simulink model "IpSDKSebesegEsPozicio"  (R2013b)
settings: Solver=FixedStepDiscrete  SolverMode=SingleTasking  StartTime=0.0  StopTime=10.0  FixedStep=1  RelTol=1e-3
undefined symbols (not defined in the file or in its folder): gcbh, xlBlockLoadCallback, xlGetNormalizedPeriod
libraries: xbsIndex_r4 x250
(part 2 of 2)

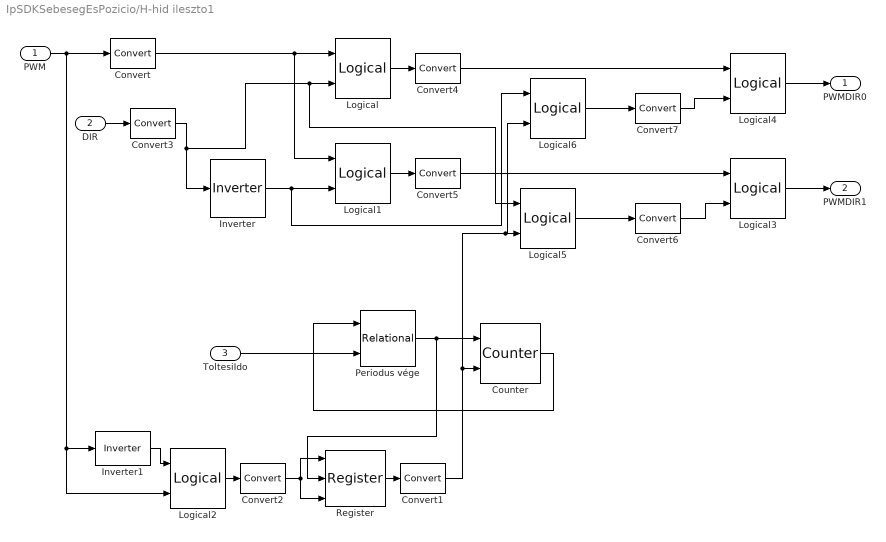
== system IpSDKSebesegEsPozicio/H-hid ileszto1 ==
  PWM : Inport
  DIR : Inport  Port=2
  ToltesiIdo : Inport  Port=3
  Convert{,1..7} (8 alike) : xbsIndex_r4/Convert  gui_display_data_type=Boolean  arith_type=Boolean  n_bits=16  bin_pt=14  float_type=Single  exp_bits=8  fraction_bits=24  quantization=Truncate  overflow=Wrap  en=off  latency=0  dbl_ovrd=off  pipeline=off  block_type=convert
  Counter : xbsIndex_r4/Counter  cnt_type=Free Running  cnt_to=Inf  operation=Up  start_count=0  cnt_by_val=1  arith_type=Unsigned  n_bits=16  bin_pt=0  load_pin=off  rst=on  en=on  explicit_period=off  period=2*10^-2  dbl_ovrd=off  use_behavioral_HDL=off  implementation=Fabric  block_type=counter
  Inverter : xbsIndex_r4/Inverter  en=off  latency=0  dbl_ovrd=off  block_type=inv
  Inverter1 : xbsIndex_r4/Inverter  en=off  latency=1  dbl_ovrd=off  block_type=inv
  Logical{,1..2,5..6} (5 alike) : xbsIndex_r4/Logical  logical_function=AND  inputs=2  en=off  latency=0  precision=User Defined  arith_type=Unsigned  n_bits=1  bin_pt=0  align_bp=on  dbl_ovrd=off  block_type=logical
  Logical3 : xbsIndex_r4/Logical  logical_function=OR  inputs=2  en=off  latency=0  precision=User Defined  arith_type=Unsigned  n_bits=1  bin_pt=0  align_bp=on  dbl_ovrd=off  block_type=logical
  Logical4 : xbsIndex_r4/Logical  logical_function=OR  inputs=2  en=off  latency=0  precision=User Defined  arith_type=Unsigned  n_bits=1  bin_pt=0  align_bp=on  dbl_ovrd=off  block_type=logical
  Periodus vége : xbsIndex_r4/Relational  mode=a=b  en=off  latency=0  dbl_ovrd=off  block_type=relational
  Register : xbsIndex_r4/Register  init=0  rst=on  en=on  dbl_ovrd=off  block_type=register
  PWMDIR0 : Outport
  PWMDIR1 : Outport  Port=2
  wires:
  DIR/1 -> Convert3/1
  Inverter/1 -> Logical6/1, Logical1/2
  Convert/1 -> Logical1/1, Logical/1
  Counter/1 -> Periodus vége/1
  Periodus vége/1 -> Register/2, Counter/1
  ToltesiIdo/1 -> Periodus vége/2
  PWM/1 -> Convert/1, Logical2/2, Inverter1/1
  Inverter1/1 -> Logical2/1
  Logical2/1 -> Convert2/1
  Logical3/1 -> PWMDIR1/1
  Logical1/1 -> Convert5/1
  Logical4/1 -> PWMDIR0/1
  Logical/1 -> Convert4/1
  Register/1 -> Convert1/1
  Convert1/1 -> Logical6/2, Logical5/2, Counter/2
  Convert2/1 -> Register/3, Register/1
  Convert3/1 -> Inverter/1, Logical5/1, Logical/2
  Convert4/1 -> Logical4/1
  Convert5/1 -> Logical3/1
  Logical5/1 -> Convert6/1
  Logical6/1 -> Convert7/1
  Convert6/1 -> Logical3/2
  Convert7/1 -> Logical4/2

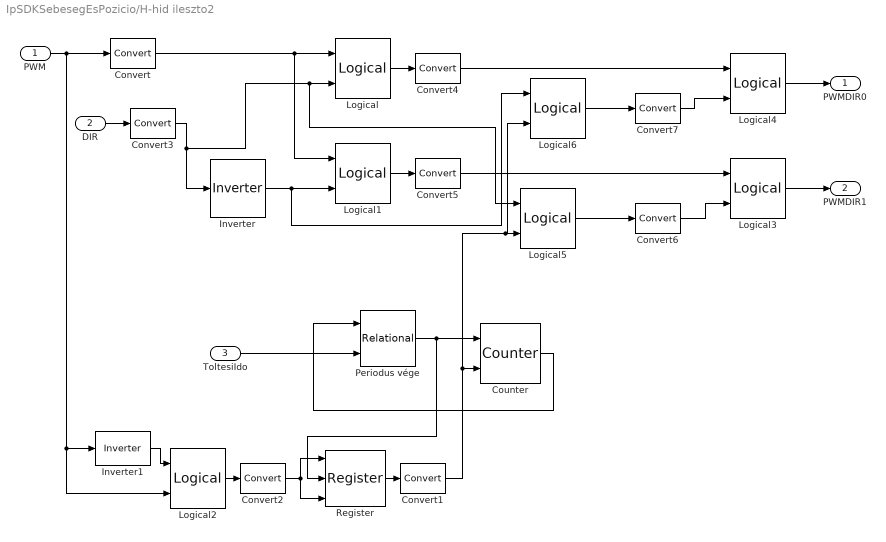
== system IpSDKSebesegEsPozicio/H-hid ileszto2 ==
  PWM : Inport
  DIR : Inport  Port=2
  ToltesiIdo : Inport  Port=3
  Convert{,1..7} (8 alike) : xbsIndex_r4/Convert  gui_display_data_type=Boolean  arith_type=Boolean  n_bits=16  bin_pt=14  float_type=Single  exp_bits=8  fraction_bits=24  quantization=Truncate  overflow=Wrap  en=off  latency=0  dbl_ovrd=off  pipeline=off  block_type=convert
  Counter : xbsIndex_r4/Counter  cnt_type=Free Running  cnt_to=Inf  operation=Up  start_count=0  cnt_by_val=1  arith_type=Unsigned  n_bits=16  bin_pt=0  load_pin=off  rst=on  en=on  explicit_period=off  period=2*10^-2  dbl_ovrd=off  use_behavioral_HDL=off  implementation=Fabric  block_type=counter
  Inverter : xbsIndex_r4/Inverter  en=off  latency=0  dbl_ovrd=off  block_type=inv
  Inverter1 : xbsIndex_r4/Inverter  en=off  latency=1  dbl_ovrd=off  block_type=inv
  Logical{,1..2,5..6} (5 alike) : xbsIndex_r4/Logical  logical_function=AND  inputs=2  en=off  latency=0  precision=User Defined  arith_type=Unsigned  n_bits=1  bin_pt=0  align_bp=on  dbl_ovrd=off  block_type=logical
  Logical3 : xbsIndex_r4/Logical  logical_function=OR  inputs=2  en=off  latency=0  precision=User Defined  arith_type=Unsigned  n_bits=1  bin_pt=0  align_bp=on  dbl_ovrd=off  block_type=logical
  Logical4 : xbsIndex_r4/Logical  logical_function=OR  inputs=2  en=off  latency=0  precision=User Defined  arith_type=Unsigned  n_bits=1  bin_pt=0  align_bp=on  dbl_ovrd=off  block_type=logical
  Periodus vége : xbsIndex_r4/Relational  mode=a=b  en=off  latency=0  dbl_ovrd=off  block_type=relational
  Register : xbsIndex_r4/Register  init=0  rst=on  en=on  dbl_ovrd=off  block_type=register
  PWMDIR0 : Outport
  PWMDIR1 : Outport  Port=2
  wires:
  DIR/1 -> Convert3/1
  Inverter/1 -> Logical6/1, Logical1/2
  Convert/1 -> Logical1/1, Logical/1
  Counter/1 -> Periodus vége/1
  Periodus vége/1 -> Register/2, Counter/1
  ToltesiIdo/1 -> Periodus vége/2
  PWM/1 -> Convert/1, Logical2/2, Inverter1/1
  Inverter1/1 -> Logical2/1
  Logical2/1 -> Convert2/1
  Logical3/1 -> PWMDIR1/1
  Logical1/1 -> Convert5/1
  Logical4/1 -> PWMDIR0/1
  Logical/1 -> Convert4/1
  Register/1 -> Convert1/1
  Convert1/1 -> Logical6/2, Logical5/2, Counter/2
  Convert2/1 -> Register/3, Register/1
  Convert3/1 -> Inverter/1, Logical5/1, Logical/2
  Convert4/1 -> Logical4/1
  Convert5/1 -> Logical3/1
  Logical5/1 -> Convert6/1
  Logical6/1 -> Convert7/1
  Convert6/1 -> Logical3/2
  Convert7/1 -> Logical4/2

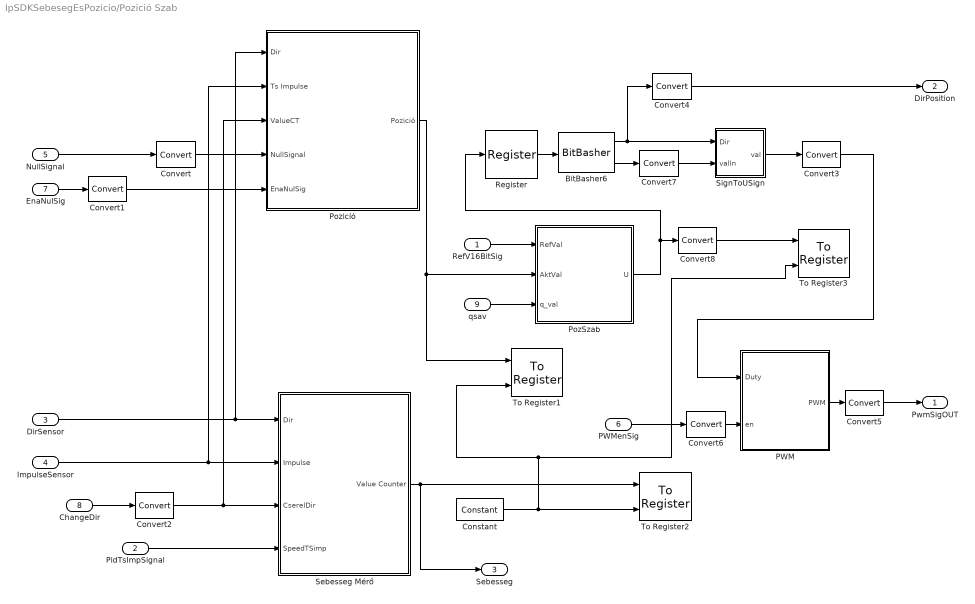
== system IpSDKSebesegEsPozicio/Pozició Szab ==
  RefV16BitSig : Inport
  PidTsImpSignal : Inport  Port=2
  DirSensor : Inport  Port=3
  ImpulseSensor : Inport  Port=4
  NullSignal : Inport  Port=5
  PWMenSig : Inport  Port=6
  EnaNulSig : Inport  Port=7
  ChangeDir : Inport  Port=8
  qsav : Inport  Port=9
  BitBasher6 : xbsIndex_r4/BitBasher  bitexpr=|  display_expr=off  sr_1=1  arith_type1=Unsigned  bin_pt1=0  sr_2=2  arith_type2="Signed  (2's comp)"  bin_pt2=0  sr_3=3  arith_type3=Unsigned  bin_pt3=0  sr_4=4  arith_type4=Unsigned  bin_pt4=0  dbl_ovrd=off  block_type=bitbasher
      | <!DOCTYPE HTML PUBLIC "-//W3C//DTD HTML 4.0//EN" "http://www.w3.org/TR/REC-html40/strict.dtd">
      | <html><head><meta name="qrichtext" content="1" /><style type="text/css">
      | p, li { white-space: pre-wrap; }
      | </style></head><body style=" font-family:'MS Shell Dlg 2'; font-size:8.25pt; font-weight:400; font-style:normal;">
      | <p style=" margin-top:12px; margin-bottom:12px; margin-left:0px; margin-right:0px; -qt-block-indent:0; text-indent:0px;"><span style=" font-family:'MS Shell Dlg'; font-size:8pt;">dir={a[16]}<br />val={a[15:0]}</span></p></body></html>
  Constant : xbsIndex_r4/Constant  const=1  gui_display_data_type=Boolean  arith_type=Boolean  n_bits=16  bin_pt=14  preci_type=Single  exp_width=8  frac_width=24  explicit_period=off  period=1  equ=P=C  opselect=C  inp2=PCIN>>17  opr=+  inp1=P  carry=CIN  dbl_ovrd=off  block_type=constant
  Convert{,1..2,6} (4 alike) : xbsIndex_r4/Convert  gui_display_data_type=Boolean  arith_type=Boolean  n_bits=16  bin_pt=14  float_type=Single  exp_bits=8  fraction_bits=24  quantization=Truncate  overflow=Wrap  en=off  latency=0  dbl_ovrd=off  pipeline=off  block_type=convert
  Convert3 : xbsIndex_r4/Convert  gui_display_data_type=Fixed-point  arith_type=Unsigned  n_bits=16  bin_pt=0  float_type=Single  exp_bits=8  fraction_bits=24  quantization=Truncate  overflow=Wrap  en=off  latency=0  dbl_ovrd=off  pipeline=off  block_type=convert
  Convert4 : xbsIndex_r4/Convert  gui_display_data_type=Boolean  arith_type=Boolean  n_bits=16  bin_pt=0  float_type=Single  exp_bits=8  fraction_bits=24  quantization=Truncate  overflow=Wrap  en=off  latency=0  dbl_ovrd=off  pipeline=off  block_type=convert
  Convert5 : xbsIndex_r4/Convert  gui_display_data_type=Boolean  arith_type=Boolean  n_bits=17  bin_pt=0  float_type=Single  exp_bits=8  fraction_bits=24  quantization=Truncate  overflow=Wrap  en=off  latency=0  dbl_ovrd=off  pipeline=off  block_type=convert
  Convert7 : xbsIndex_r4/Convert  gui_display_data_type=Fixed-point  arith_type=Unsigned  n_bits=16  bin_pt=0  float_type=Single  exp_bits=8  fraction_bits=24  quantization=Truncate  overflow=Wrap  en=off  latency=0  dbl_ovrd=off  pipeline=off  block_type=convert
  Convert8 : xbsIndex_r4/Convert  gui_display_data_type=Fixed-point  arith_type="Signed  (2's comp)"  n_bits=32  bin_pt=0  float_type=Single  exp_bits=8  fraction_bits=24  quantization=Truncate  overflow=Wrap  en=off  latency=0  dbl_ovrd=off  pipeline=off  block_type=convert
  PWM : Subsystem
  PozSzab : Subsystem
  Pozicíó : Subsystem
  Register : xbsIndex_r4/Register  init=0  rst=off  en=off  dbl_ovrd=off  block_type=register
  Sebesseg Mérő : Subsystem
  SignToUSign : Subsystem
  To Register1 : xbsIndex_r4/To Register  shared_memory_name='AktPozicio'  init=0  ownership=Locally owned and initialized  explicit_data_type=on  gui_display_data_type=Fixed-point  arith_type="Signed  (2's comp)"  n_bits=16  bin_pt=0  preci_type=Single  dbl_ovrd=off  block_type=toreg
      settings: AttributesFormatString=<< %<shared_memory_name> >>  infoedit="Register block that writes data to a shared memory register.  Delay of one sample period."
  To Register2 : xbsIndex_r4/To Register  shared_memory_name='SebessegPozicio'  init=0  ownership=Locally owned and initialized  explicit_data_type=on  gui_display_data_type=Fixed-point  arith_type="Signed  (2's comp)"  n_bits=16  bin_pt=0  preci_type=Single  dbl_ovrd=off  block_type=toreg
      settings: AttributesFormatString=<< %<shared_memory_name> >>  infoedit="Register block that writes data to a shared memory register.  Delay of one sample period."
  To Register3 : xbsIndex_r4/To Register  shared_memory_name='UPozicio'  init=0  ownership=Locally owned and initialized  explicit_data_type=on  gui_display_data_type=Fixed-point  arith_type="Signed  (2's comp)"  n_bits=32  bin_pt=0  preci_type=Single  dbl_ovrd=off  block_type=toreg
      settings: AttributesFormatString=<< %<shared_memory_name> >>  infoedit="Register block that writes data to a shared memory register.  Delay of one sample period."  xl_use_area=on  xl_area=[100,0,0,0,0,0,0]
  PwmSigOUT : Outport
  DirPosition : Outport  Port=2
  Sebesseg : Outport  Port=3
  wires:
  PWM/1(PWM) -> Convert5/1
  BitBasher6/1 -> SignToUSign/1(Dir), Convert4/1
  BitBasher6/2 -> Convert7/1
  SignToUSign/1(val) -> Convert3/1
  PozSzab/1(U) -> Register/1, Convert8/1
  Convert3/1 -> PWM/1(Duty)
  Convert7/1 -> SignToUSign/2(valIn)
  RefV16BitSig/1 -> PozSzab/1(RefVal)
  PWMenSig/1 -> Convert6/1
  Convert5/1 -> PwmSigOUT/1
  NullSignal/1 -> Convert/1
  EnaNulSig/1 -> Convert1/1
  Convert4/1 -> DirPosition/1
  ChangeDir/1 -> Convert2/1
  Pozicíó/1(Pozició) -> To Register1/1, PozSzab/2(AktVal)
  qsav/1 -> PozSzab/3(q_val)
  Sebesseg Mérő/1(Value Counter) -> To Register2/1, Sebesseg/1
  Constant/1 -> To Register3/2, To Register1/2, To Register2/2
  Convert8/1 -> To Register3/1
  PidTsImpSignal/1 -> Sebesseg Mérő/4(SpeedTSimp)
  Register/1 -> BitBasher6/1
  Convert/1 -> Pozicíó/4(NullSignal)
  Convert1/1 -> Pozicíó/5(EnaNulSig)
  DirSensor/1 -> Pozicíó/1(Dir), Sebesseg Mérő/1(Dir)
  ImpulseSensor/1 -> Pozicíó/2(Ts Impulse), Sebesseg Mérő/2(Impulse)
  Convert2/1 -> Pozicíó/3(ValueCT), Sebesseg Mérő/3(CserelDir)
  Convert6/1 -> PWM/2(en)

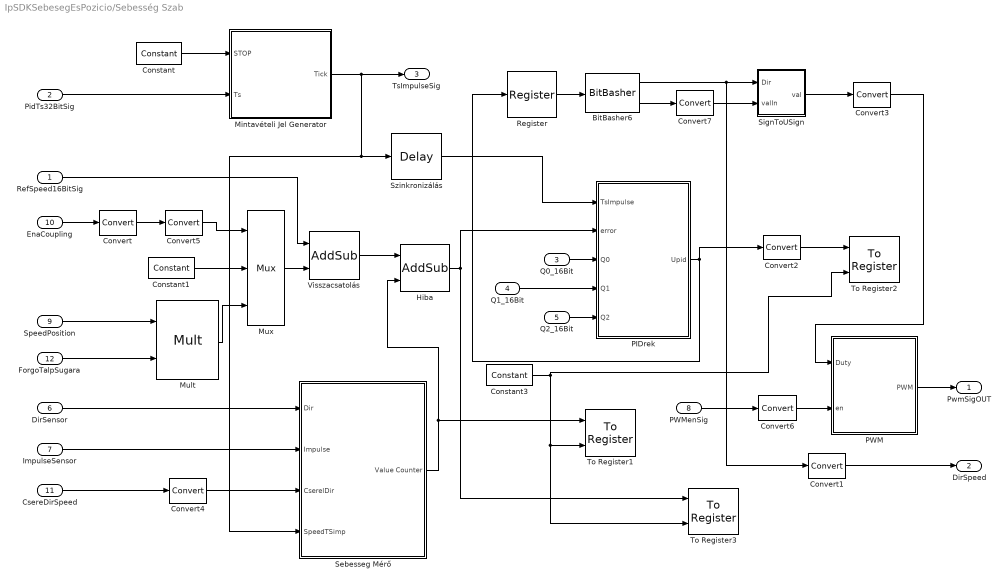
== system IpSDKSebesegEsPozicio/Sebesség Szab ==
  RefSpeed16BitSig : Inport
  PidTs32BitSig : Inport  Port=2
  Q0_16Bit : Inport  Port=3
  Q1_16Bit : Inport  Port=4
  Q2_16Bit : Inport  Port=5
  DirSensor : Inport  Port=6
  ImpulseSensor : Inport  Port=7
  PWMenSig : Inport  Port=8
  SpeedPosition : Inport  Port=9
  EnaCoupling : Inport  Port=10
  CsereDirSpeed : Inport  Port=11
  ForgoTalpSugara : Inport  Port=12
  BitBasher6 : xbsIndex_r4/BitBasher  bitexpr=|  display_expr=off  sr_1=1  arith_type1=Unsigned  bin_pt1=0  sr_2=2  arith_type2=Unsigned  bin_pt2=0  sr_3=3  arith_type3=Unsigned  bin_pt3=0  sr_4=4  arith_type4=Unsigned  bin_pt4=0  dbl_ovrd=off  block_type=bitbasher
      | <!DOCTYPE HTML PUBLIC "-//W3C//DTD HTML 4.0//EN" "http://www.w3.org/TR/REC-html40/strict.dtd">
      | <html><head><meta name="qrichtext" content="1" /><style type="text/css">
      | p, li { white-space: pre-wrap; }
      | </style></head><body style=" font-family:'MS Shell Dlg 2'; font-size:8.25pt; font-weight:400; font-style:normal;">
      | <p style=" margin-top:12px; margin-bottom:12px; margin-left:0px; margin-right:0px; -qt-block-indent:0; text-indent:0px;"><span style=" font-family:'MS Shell Dlg'; font-size:8pt;">dir={a[16]}<br />val={a[15:0]}</span></p></body></html>
  Constant : xbsIndex_r4/Constant  const=0  gui_display_data_type=Boolean  arith_type=Boolean  n_bits=16  bin_pt=14  preci_type=Single  exp_width=8  frac_width=24  explicit_period=off  period=1  equ=P=C  opselect=C  inp2=PCIN>>17  opr=+  inp1=P  carry=CIN  dbl_ovrd=off  block_type=constant
  Constant1 : xbsIndex_r4/Constant  const=0  gui_display_data_type=Fixed-point  arith_type=Signed (2's comp)  n_bits=16  bin_pt=0  preci_type=Single  exp_width=8  frac_width=24  explicit_period=off  period=1  equ=P=C  opselect=C  inp2=PCIN>>17  opr=+  inp1=P  carry=CIN  dbl_ovrd=off  block_type=constant
  Constant3 : xbsIndex_r4/Constant  const=1  gui_display_data_type=Boolean  arith_type=Boolean  n_bits=16  bin_pt=14  preci_type=Single  exp_width=8  frac_width=24  explicit_period=off  period=1  equ=P=C  opselect=C  inp2=PCIN>>17  opr=+  inp1=P  carry=CIN  dbl_ovrd=off  block_type=constant
  Convert{,4..6} (4 alike) : xbsIndex_r4/Convert  gui_display_data_type=Boolean  arith_type=Boolean  n_bits=16  bin_pt=14  float_type=Single  exp_bits=8  fraction_bits=24  quantization=Truncate  overflow=Wrap  en=off  latency=0  dbl_ovrd=off  pipeline=off  block_type=convert
  Convert1 : xbsIndex_r4/Convert  gui_display_data_type=Boolean  arith_type=Boolean  n_bits=16  bin_pt=0  float_type=Single  exp_bits=8  fraction_bits=24  quantization=Truncate  overflow=Wrap  en=off  latency=0  dbl_ovrd=off  pipeline=off  block_type=convert
  Convert2 : xbsIndex_r4/Convert  gui_display_data_type=Fixed-point  arith_type="Signed  (2's comp)"  n_bits=32  bin_pt=0  float_type=Single  exp_bits=8  fraction_bits=24  quantization=Truncate  overflow=Saturate  en=off  latency=0  dbl_ovrd=off  pipeline=off  block_type=convert
  Convert3 : xbsIndex_r4/Convert  gui_display_data_type=Fixed-point  arith_type=Unsigned  n_bits=16  bin_pt=0  float_type=Single  exp_bits=8  fraction_bits=24  quantization=Truncate  overflow=Wrap  en=off  latency=0  dbl_ovrd=off  pipeline=off  block_type=convert
  Convert7 : xbsIndex_r4/Convert  gui_display_data_type=Fixed-point  arith_type=Unsigned  n_bits=16  bin_pt=0  float_type=Single  exp_bits=8  fraction_bits=24  quantization=Truncate  overflow=Wrap  en=off  latency=0  dbl_ovrd=off  pipeline=off  block_type=convert
  Hiba : xbsIndex_r4/AddSub  mode=Subtraction  use_carryin=off  use_carryout=off  en=off  latency=0  precision=User Defined  arith_type="Signed  (2's comp)"  n_bits=16  bin_pt=0  quantization=Truncate  overflow=Saturate  dbl_ovrd=off  use_behavioral_HDL=off  hw_selection=Fabric  pipelined=off  block_type=addsub
      settings: xl_area=[10,0,0,0,0,0,0]
  Mintavételi Jel Generator : Subsystem
  Mult : xbsIndex_r4/Mult  precision=User Defined  arith_type="Signed  (2's comp)"  n_bits=16  bin_pt=0  quantization=Truncate  overflow=Saturate  en=off  latency=3  dbl_ovrd=off  use_behavioral_HDL=off  opt=Area  use_embedded=on  optimum_pipeline=off  pipeline=on  use_rpm=on  placement_style=Triangular  block_type=mult
  Mux : xbsIndex_r4/Mux  inputs=2  en=off  latency=0  precision=User Defined  arith_type="Signed  (2's comp)"  n_bits=16  bin_pt=0  quantization=Truncate  overflow=Saturate  dbl_ovrd=off  block_type=mux
      settings: xl_use_area=on  xl_area=[1,0,0,0,0,0,0]
  PIDrek : Subsystem
  PWM : Subsystem
  Register : xbsIndex_r4/Register  init=0  rst=off  en=off  dbl_ovrd=off  block_type=register
  Sebesseg Mérő : Subsystem
  SignToUSign : Subsystem
  Szinkronizálás : xbsIndex_r4/Delay  rst=off  infoeditControl=Selection of Reset will increase slice count due to use of real FFs and instead of SRLs  en=off  latency=6  dbl_ovrd=off  reg_retiming=off  block_type=delay
      settings: xl_area=[10,0,0,0,0,0,0]
  To Register1 : xbsIndex_r4/To Register  shared_memory_name='AktSebesseg'  init=0  ownership=Locally owned and initialized  explicit_data_type=on  gui_display_data_type=Fixed-point  arith_type="Signed  (2's comp)"  n_bits=16  bin_pt=0  preci_type=Single  dbl_ovrd=off  block_type=toreg
      settings: AttributesFormatString=<< %<shared_memory_name> >>  infoedit="Register block that writes data to a shared memory register.  Delay of one sample period."
  To Register2 : xbsIndex_r4/To Register  shared_memory_name='USebesseg'  init=0  ownership=Locally owned and initialized  explicit_data_type=on  gui_display_data_type=Fixed-point  arith_type="Signed  (2's comp)"  n_bits=32  bin_pt=0  preci_type=Single  dbl_ovrd=off  block_type=toreg
      settings: AttributesFormatString=<< %<shared_memory_name> >>  infoedit="Register block that writes data to a shared memory register.  Delay of one sample period."
  To Register3 : xbsIndex_r4/To Register  shared_memory_name='eSebesseg'  init=0  ownership=Locally owned and initialized  explicit_data_type=on  gui_display_data_type=Fixed-point  arith_type="Signed  (2's comp)"  n_bits=16  bin_pt=0  preci_type=Single  dbl_ovrd=off  block_type=toreg
      settings: AttributesFormatString=<< %<shared_memory_name> >>  infoedit="Register block that writes data to a shared memory register.  Delay of one sample period."
  Visszacsatolás : xbsIndex_r4/AddSub  mode=Subtraction  use_carryin=off  use_carryout=off  en=off  latency=0  precision=User Defined  arith_type="Signed  (2's comp)"  n_bits=16  bin_pt=0  quantization=Truncate  overflow=Saturate  dbl_ovrd=off  use_behavioral_HDL=off  hw_selection=Fabric  pipelined=off  block_type=addsub
  PwmSigOUT : Outport
  DirSpeed : Outport  Port=2
  TsImpulseSig : Outport  Port=3
  wires:
  BitBasher6/1 -> SignToUSign/1(Dir), Convert1/1
  BitBasher6/2 -> Convert7/1
  SignToUSign/1(val) -> Convert3/1
  PIDrek/1(Upid) -> Convert2/1, Register/1
  Convert3/1 -> PWM/1(Duty)
  Convert7/1 -> SignToUSign/2(valIn)
  Mintavételi Jel Generator/1(Tick) -> TsImpulseSig/1, Szinkronizálás/1, Sebesseg Mérő/4(SpeedTSimp)
  Constant/1 -> Mintavételi Jel Generator/1(STOP)
  Szinkronizálás/1 -> PIDrek/1(TsImpulse)
  PidTs32BitSig/1 -> Mintavételi Jel Generator/2(Ts)
  Q2_16Bit/1 -> PIDrek/5(Q2)
  Q1_16Bit/1 -> PIDrek/4(Q1)
  Q0_16Bit/1 -> PIDrek/3(Q0)
  DirSensor/1 -> Sebesseg Mérő/1(Dir)
  ImpulseSensor/1 -> Sebesseg Mérő/2(Impulse)
  PWMenSig/1 -> Convert6/1
  PWM/1(PWM) -> PwmSigOUT/1
  Convert1/1 -> DirSpeed/1
  SpeedPosition/1 -> Mult/1
  Mux/1 -> Visszacsatolás/2
  Constant1/1 -> Mux/2
  Mult/1 -> Mux/3
  EnaCoupling/1 -> Convert/1
  ForgoTalpSugara/1 -> Mult/2
  CsereDirSpeed/1 -> Convert4/1
  Sebesseg Mérő/1(Value Counter) -> Hiba/2, To Register1/1
  Constant3/1 -> To Register3/2, To Register1/2, To Register2/2
  Convert2/1 -> To Register2/1
  Hiba/1 -> To Register3/1, PIDrek/2(error)
  Register/1 -> BitBasher6/1
  RefSpeed16BitSig/1 -> Visszacsatolás/1
  Visszacsatolás/1 -> Hiba/1
  Convert4/1 -> Sebesseg Mérő/3(CserelDir)
  Convert5/1 -> Mux/1
  Convert6/1 -> PWM/2(en)
  Convert/1 -> Convert5/1

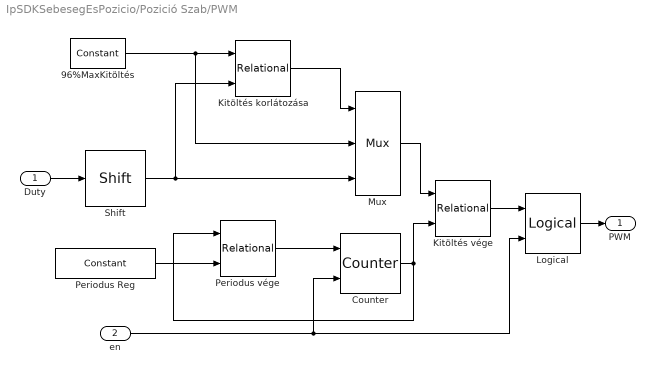
== system IpSDKSebesegEsPozicio/Pozició Szab/PWM ==
  Duty : Inport
  en : Inport  Port=2
  96%MaxKitöltés : xbsIndex_r4/Constant  const=15563  gui_display_data_type=Fixed-point  arith_type=Unsigned  n_bits=16  bin_pt=0  preci_type=Single  exp_width=8  frac_width=24  explicit_period=off  period=1  equ=P=C  opselect=C  inp2=PCIN>>17  opr=+  inp1=P  carry=CIN  dbl_ovrd=off  block_type=constant
  Counter : xbsIndex_r4/Counter  cnt_type=Free Running  cnt_to=Inf  operation=Up  start_count=0  cnt_by_val=1  arith_type=Unsigned  n_bits=16  bin_pt=0  load_pin=off  rst=on  en=on  explicit_period=off  period=2*10^-2  dbl_ovrd=off  use_behavioral_HDL=off  implementation=Fabric  block_type=counter
  Kitöltés vége : xbsIndex_r4/Relational  mode=a>b  en=off  latency=0  dbl_ovrd=off  block_type=relational
  Kitöltés korlátozása : xbsIndex_r4/Relational  mode=a>b  en=off  latency=0  dbl_ovrd=off  block_type=relational
  Logical : xbsIndex_r4/Logical  logical_function=AND  inputs=2  en=off  latency=0  precision=User Defined  arith_type=Unsigned  n_bits=1  bin_pt=0  align_bp=on  dbl_ovrd=off  block_type=logical
  Mux : xbsIndex_r4/Mux  inputs=2  en=off  latency=0  precision=User Defined  arith_type=Unsigned  n_bits=16  bin_pt=0  quantization=Truncate  overflow=Wrap  dbl_ovrd=off  block_type=mux
  Periodus vége : xbsIndex_r4/Relational  mode=a=b  en=off  latency=0  dbl_ovrd=off  block_type=relational
  Periodus Reg : xbsIndex_r4/Constant  const=16383  gui_display_data_type=Fixed-point  arith_type=Unsigned  n_bits=17  bin_pt=0  preci_type=Single  exp_width=8  frac_width=24  explicit_period=off  period=1  equ=P=C  opselect=C  inp2=PCIN>>17  opr=+  inp1=P  carry=CIN  dbl_ovrd=off  block_type=constant
  Shift : xbsIndex_r4/Shift  shift_dir=Right  shift_bits=2  en=off  latency=0  precision=User Defined  arith_type="Signed  (2's comp)"  n_bits=16  bin_pt=0  quantization=Truncate  overflow=Saturate  dbl_ovrd=off  block_type=shift
  PWM : Outport
  wires:
  Counter/1 -> Periodus vége/1, Kitöltés vége/2
  Periodus vége/1 -> Counter/1
  en/1 -> Logical/2, Counter/2
  Kitöltés vége/1 -> Logical/1
  Logical/1 -> PWM/1
  Duty/1 -> Shift/1
  Periodus Reg/1 -> Periodus vége/2
  96%MaxKitöltés/1 -> Mux/2, Kitöltés korlátozása/1
  Mux/1 -> Kitöltés vége/1
  Kitöltés korlátozása/1 -> Mux/1
  Shift/1 -> Mux/3, Kitöltés korlátozása/2

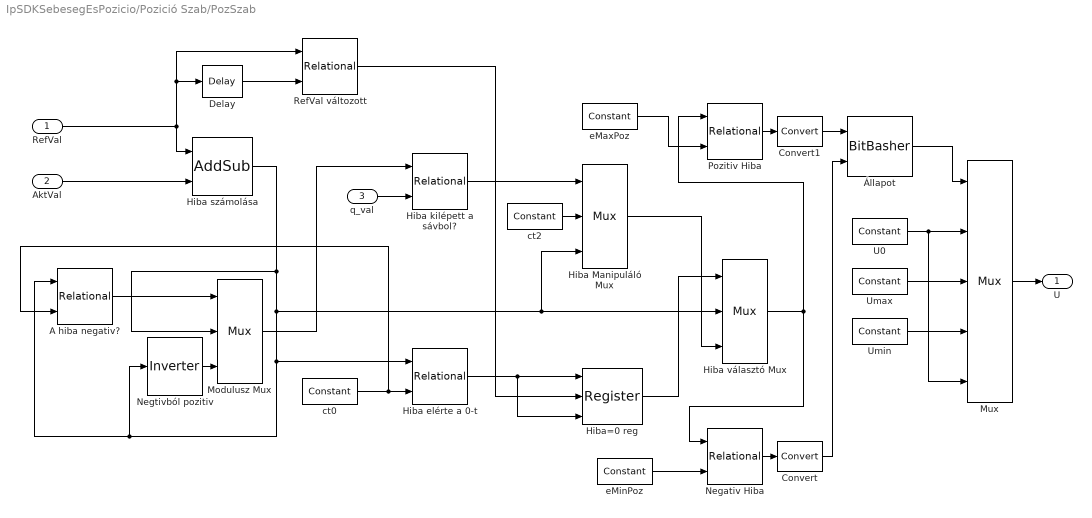
== system IpSDKSebesegEsPozicio/Pozició Szab/PozSzab ==
  RefVal : Inport
  AktVal : Inport  Port=2
  q_val : Inport  Port=3
  A hiba negativ? : xbsIndex_r4/Relational  mode=a<b  en=off  latency=0  dbl_ovrd=off  block_type=relational
  Convert : xbsIndex_r4/Convert  gui_display_data_type=Boolean  arith_type=Boolean  n_bits=16  bin_pt=14  float_type=Single  exp_bits=8  fraction_bits=24  quantization=Truncate  overflow=Wrap  en=off  latency=0  dbl_ovrd=off  pipeline=off  block_type=convert
  Convert1 : xbsIndex_r4/Convert  gui_display_data_type=Boolean  arith_type=Boolean  n_bits=16  bin_pt=14  float_type=Single  exp_bits=8  fraction_bits=24  quantization=Truncate  overflow=Wrap  en=off  latency=0  dbl_ovrd=off  pipeline=off  block_type=convert
  Delay : xbsIndex_r4/Delay  rst=off  infoeditControl=Selection of Reset will increase slice count due to use of real FFs and instead of SRLs  en=off  latency=1  dbl_ovrd=off  reg_retiming=off  block_type=delay
  Hiba elérte a 0-t : xbsIndex_r4/Relational  mode=a=b  en=off  latency=2  dbl_ovrd=off  block_type=relational
  Hiba számolása : xbsIndex_r4/AddSub  mode=Subtraction  use_carryin=off  use_carryout=off  en=off  latency=0  precision=User Defined  arith_type="Signed  (2's comp)"  n_bits=17  bin_pt=0  quantization=Truncate  overflow=Saturate  dbl_ovrd=off  use_behavioral_HDL=off  hw_selection=Fabric  pipelined=off  block_type=addsub
  Hiba Manipuláló Mux : xbsIndex_r4/Mux  inputs=2  en=off  latency=0  precision=User Defined  arith_type="Signed  (2's comp)"  n_bits=17  bin_pt=0  quantization=Truncate  overflow=Wrap  dbl_ovrd=off  block_type=mux
  Hiba kilépett a sávbol? : xbsIndex_r4/Relational  mode=a>=b  en=off  latency=0  dbl_ovrd=off  block_type=relational
  Hiba választó Mux : xbsIndex_r4/Mux  inputs=2  en=off  latency=0  precision=User Defined  arith_type="Signed  (2's comp)"  n_bits=17  bin_pt=0  quantization=Truncate  overflow=Wrap  dbl_ovrd=off  block_type=mux
      settings: xl_use_area=on  xl_area=[200,0,0,0,0,0,0]
  Hiba=0 reg : xbsIndex_r4/Register  init=0  rst=on  en=on  dbl_ovrd=off  block_type=register
  Modulusz Mux : xbsIndex_r4/Mux  inputs=2  en=off  latency=0  precision=User Defined  arith_type="Signed  (2's comp)"  n_bits=17  bin_pt=0  quantization=Truncate  overflow=Wrap  dbl_ovrd=off  block_type=mux
  Mux : xbsIndex_r4/Mux  inputs=4  en=off  latency=0  precision=User Defined  arith_type="Signed  (2's comp)"  n_bits=17  bin_pt=0  quantization=Truncate  overflow=Wrap  dbl_ovrd=off  block_type=mux
      settings: xl_use_area=on  xl_area=[1000,0,0,0,0,0,0]
  Negativ Hiba : xbsIndex_r4/Relational  mode=a<=b  en=off  latency=0  dbl_ovrd=off  block_type=relational
  Negtivból pozitiv : xbsIndex_r4/Inverter  en=off  latency=0  dbl_ovrd=off  block_type=inv
  Pozitiv Hiba : xbsIndex_r4/Relational  mode=a>=b  en=off  latency=0  dbl_ovrd=off  block_type=relational
      settings: xl_use_area=on  xl_area=[100,0,0,0,0,0,0]
  RefVal változott : xbsIndex_r4/Relational  mode=a!=b  en=off  latency=0  dbl_ovrd=off  block_type=relational
  U0 : xbsIndex_r4/Constant  const=0  gui_display_data_type=Fixed-point  arith_type=Signed (2's comp)  n_bits=17  bin_pt=0  preci_type=Single  exp_width=8  frac_width=24  explicit_period=off  period=1  equ=P=C  opselect=C  inp2=PCIN>>17  opr=+  inp1=P  carry=CIN  dbl_ovrd=off  block_type=constant
  Umax : xbsIndex_r4/Constant  const=64000  gui_display_data_type=Fixed-point  arith_type=Signed (2's comp)  n_bits=17  bin_pt=0  preci_type=Single  exp_width=8  frac_width=24  explicit_period=on  period=1  equ=P=C  opselect=C  inp2=PCIN>>17  opr=+  inp1=P  carry=CIN  dbl_ovrd=off  block_type=constant
  Umin : xbsIndex_r4/Constant  const=-64000  gui_display_data_type=Fixed-point  arith_type=Signed (2's comp)  n_bits=17  bin_pt=0  preci_type=Single  exp_width=8  frac_width=24  explicit_period=on  period=1  equ=P=C  opselect=C  inp2=PCIN>>17  opr=+  inp1=P  carry=CIN  dbl_ovrd=off  block_type=constant
  ct0 : xbsIndex_r4/Constant  const=0  gui_display_data_type=Fixed-point  arith_type=Signed (2's comp)  n_bits=17  bin_pt=0  preci_type=Single  exp_width=8  frac_width=24  explicit_period=off  period=1  equ=P=C  opselect=C  inp2=PCIN>>17  opr=+  inp1=P  carry=CIN  dbl_ovrd=off  block_type=constant
  ct2 : xbsIndex_r4/Constant  const=0  gui_display_data_type=Fixed-point  arith_type=Signed (2's comp)  n_bits=17  bin_pt=0  preci_type=Single  exp_width=8  frac_width=24  explicit_period=off  period=1  equ=P=C  opselect=C  inp2=PCIN>>17  opr=+  inp1=P  carry=CIN  dbl_ovrd=off  block_type=constant
  eMaxPoz : xbsIndex_r4/Constant  const=1  gui_display_data_type=Fixed-point  arith_type=Signed (2's comp)  n_bits=17  bin_pt=0  preci_type=Single  exp_width=8  frac_width=24  explicit_period=on  period=1  equ=P=C  opselect=C  inp2=PCIN>>17  opr=+  inp1=P  carry=CIN  dbl_ovrd=off  block_type=constant
  eMinPoz : xbsIndex_r4/Constant  const=-1  gui_display_data_type=Fixed-point  arith_type=Signed (2's comp)  n_bits=17  bin_pt=0  preci_type=Single  exp_width=8  frac_width=24  explicit_period=on  period=1  equ=P=C  opselect=C  inp2=PCIN>>17  opr=+  inp1=P  carry=CIN  dbl_ovrd=off  block_type=constant
  Állapot : xbsIndex_r4/BitBasher  bitexpr=|  display_expr=off  sr_1=1  arith_type1=Unsigned  bin_pt1=0  sr_2=2  arith_type2=Unsigned  bin_pt2=0  sr_3=3  arith_type3=Unsigned  bin_pt3=0  sr_4=4  arith_type4=Unsigned  bin_pt4=0  dbl_ovrd=off  block_type=bitbasher
      | <!DOCTYPE HTML PUBLIC "-//W3C//DTD HTML 4.0//EN" "http://www.w3.org/TR/REC-html40/strict.dtd">
      | <html><head><meta name="qrichtext" content="1" /><style type="text/css">
      | p, li { white-space: pre-wrap; }
      | </style></head><body style=" font-family:'MS Shell Dlg 2'; font-size:8.25pt; font-weight:400; font-style:normal;">
      | <p style=" margin-top:12px; margin-bottom:12px; margin-left:0px; margin-right:0px; -qt-block-indent:0; text-indent:0px;"><span style=" font-family:'MS Shell Dlg'; font-size:8pt;">a={b,c}</span></p></body></html>
  U : Outport
  wires:
  Mux/1 -> U/1
  eMaxPoz/1 -> Pozitiv Hiba/2
  eMinPoz/1 -> Negativ Hiba/2
  Pozitiv Hiba/1 -> Convert1/1
  Negativ Hiba/1 -> Convert/1
  Convert/1 -> Állapot/2
  Állapot/1 -> Mux/1
  Convert1/1 -> Állapot/1
  Umin/1 -> Mux/4
  U0/1 -> Mux/5, Mux/2
  Hiba kilépett a sávbol?/1 -> Hiba Manipuláló Mux/1
  Modulusz Mux/1 -> Hiba kilépett a sávbol?/1
  q_val/1 -> Hiba kilépett a sávbol?/2
  ct2/1 -> Hiba Manipuláló Mux/2
  Hiba választó Mux/1 -> Negativ Hiba/1, Pozitiv Hiba/1
  Hiba elérte a 0-t/1 -> Hiba=0 reg/1, Hiba=0 reg/3
  Hiba Manipuláló Mux/1 -> Hiba választó Mux/3
  Delay/1 -> RefVal változott/2
  RefVal/1 -> Hiba számolása/1, RefVal változott/1, Delay/1
  RefVal változott/1 -> Hiba=0 reg/2
  AktVal/1 -> Hiba számolása/2
  Umax/1 -> Mux/3
  Hiba=0 reg/1 -> Hiba választó Mux/1
  Hiba számolása/1 -> Negtivból pozitiv/1, A hiba negativ?/1, Hiba elérte a 0-t/1, Hiba választó Mux/2, Hiba Manipuláló Mux/3, Modulusz Mux/2
  Negtivból pozitiv/1 -> Modulusz Mux/3
  A hiba negativ?/1 -> Modulusz Mux/1
  ct0/1 -> A hiba negativ?/2, Hiba elérte a 0-t/2

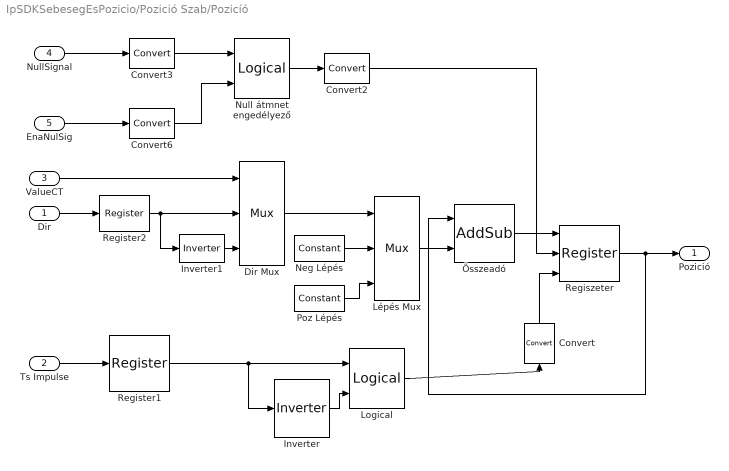
== system IpSDKSebesegEsPozicio/Pozició Szab/Pozicíó ==
  Dir : Inport
  Ts Impulse : Inport  Port=2
  ValueCT : Inport  Port=3
  NullSignal : Inport  Port=4
  EnaNulSig : Inport  Port=5
  Convert : xbsIndex_r4/Convert  gui_display_data_type=Boolean  arith_type=Boolean  n_bits=16  bin_pt=14  float_type=Single  exp_bits=8  fraction_bits=24  quantization=Truncate  overflow=Wrap  en=off  latency=0  dbl_ovrd=off  pipeline=off  block_type=convert
  Convert2 : xbsIndex_r4/Convert  gui_display_data_type=Boolean  arith_type=Boolean  n_bits=1  bin_pt=0  float_type=Single  exp_bits=8  fraction_bits=24  quantization=Truncate  overflow=Wrap  en=off  latency=0  dbl_ovrd=off  pipeline=off  block_type=convert
  Convert3 : xbsIndex_r4/Convert  gui_display_data_type=Boolean  arith_type=Boolean  n_bits=17  bin_pt=0  float_type=Single  exp_bits=8  fraction_bits=24  quantization=Truncate  overflow=Wrap  en=off  latency=0  dbl_ovrd=off  pipeline=off  block_type=convert
  Convert6 : xbsIndex_r4/Convert  gui_display_data_type=Boolean  arith_type=Boolean  n_bits=17  bin_pt=0  float_type=Single  exp_bits=8  fraction_bits=24  quantization=Truncate  overflow=Wrap  en=off  latency=0  dbl_ovrd=off  pipeline=off  block_type=convert
  Dir Mux : xbsIndex_r4/Mux  inputs=2  en=off  latency=0  precision=User Defined  arith_type=Unsigned  n_bits=1  bin_pt=0  quantization=Truncate  overflow=Saturate  dbl_ovrd=off  block_type=mux
  Inverter : xbsIndex_r4/Inverter  en=off  latency=1  dbl_ovrd=off  block_type=inv
  Inverter1 : xbsIndex_r4/Inverter  en=off  latency=0  dbl_ovrd=off  block_type=inv
  Logical : xbsIndex_r4/Logical  logical_function=AND  inputs=2  en=off  latency=0  precision=Full  arith_type=Unsigned  n_bits=16  bin_pt=0  align_bp=on  dbl_ovrd=off  block_type=logical
  Lépés Mux : xbsIndex_r4/Mux  inputs=2  en=off  latency=0  precision=User Defined  arith_type="Signed  (2's comp)"  n_bits=16  bin_pt=0  quantization=Truncate  overflow=Saturate  dbl_ovrd=off  block_type=mux
  Neg Lépés : xbsIndex_r4/Constant  const=-1  gui_display_data_type=Fixed-point  arith_type=Signed (2's comp)  n_bits=16  bin_pt=0  preci_type=Single  exp_width=8  frac_width=24  explicit_period=off  period=1  equ=P=C  opselect=C  inp2=PCIN>>17  opr=+  inp1=P  carry=CIN  dbl_ovrd=off  block_type=constant
  Null átmnet engedélyező : xbsIndex_r4/Logical  logical_function=AND  inputs=2  en=off  latency=0  precision=Full  arith_type="Signed  (2's comp)"  n_bits=1  bin_pt=0  align_bp=on  dbl_ovrd=off  block_type=logical
  Poz Lépés : xbsIndex_r4/Constant  const=1  gui_display_data_type=Fixed-point  arith_type=Signed (2's comp)  n_bits=16  bin_pt=0  preci_type=Single  exp_width=8  frac_width=24  explicit_period=off  period=1  equ=P=C  opselect=C  inp2=PCIN>>17  opr=+  inp1=P  carry=CIN  dbl_ovrd=off  block_type=constant
  Register1 : xbsIndex_r4/Register  init=0  rst=off  en=off  dbl_ovrd=off  block_type=register
  Register2 : xbsIndex_r4/Register  init=0  rst=off  en=off  dbl_ovrd=off  block_type=register
  Regiszeter : xbsIndex_r4/Register  init=0  rst=on  en=on  dbl_ovrd=off  block_type=register
      settings: xl_use_area=on  xl_area=[100,0,0,0,0,0,0]
  Összeadó : xbsIndex_r4/AddSub  mode=Addition  use_carryin=off  use_carryout=off  en=off  latency=0  precision=User Defined  arith_type="Signed  (2's comp)"  n_bits=16  bin_pt=0  quantization=Truncate  overflow=Saturate  dbl_ovrd=off  use_behavioral_HDL=off  hw_selection=Fabric  pipelined=off  block_type=addsub
  Pozició : Outport
  wires:
  Poz Lépés/1 -> Lépés Mux/3
  Dir/1 -> Register2/1
  Inverter/1 -> Logical/2
  Logical/1 -> Convert/1
  Ts Impulse/1 -> Register1/1
  Regiszeter/1 -> Pozició/1, Összeadó/1
  Convert/1 -> Regiszeter/3
  Convert2/1 -> Regiszeter/2
  Register1/1 -> Logical/1, Inverter/1
  Összeadó/1 -> Regiszeter/1
  Lépés Mux/1 -> Összeadó/2
  Neg Lépés/1 -> Lépés Mux/2
  Register2/1 -> Inverter1/1, Dir Mux/2
  Dir Mux/1 -> Lépés Mux/1
  ValueCT/1 -> Dir Mux/1
  Inverter1/1 -> Dir Mux/3
  Null átmnet engedélyező/1 -> Convert2/1
  Convert6/1 -> Null átmnet engedélyező/2
  NullSignal/1 -> Convert3/1
  EnaNulSig/1 -> Convert6/1
  Convert3/1 -> Null átmnet engedélyező/1

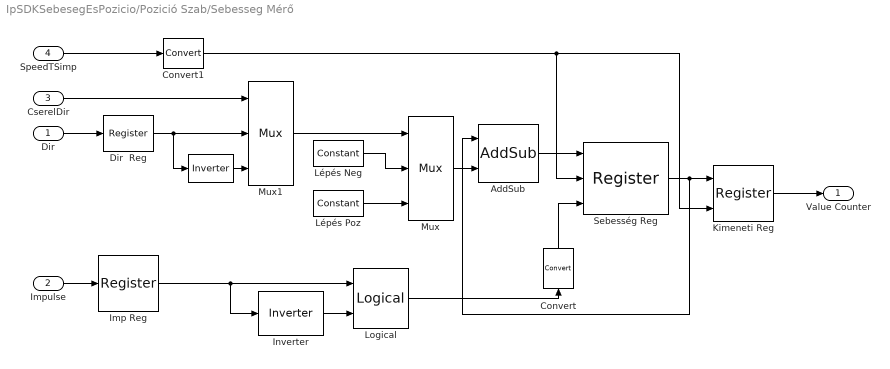
== system IpSDKSebesegEsPozicio/Pozició Szab/Sebesseg Mérő ==
  Dir : Inport
  Impulse : Inport  Port=2
  CserelDir : Inport  Port=3
  SpeedTSimp : Inport  Port=4
  " " : xbsIndex_r4/Inverter  en=off  latency=0  dbl_ovrd=off  block_type=inv
      settings: xl_area=[10,0,0,0,0,0,0]
  AddSub : xbsIndex_r4/AddSub  mode=Addition  use_carryin=off  use_carryout=off  en=off  latency=0  precision=User Defined  arith_type="Signed  (2's comp)"  n_bits=16  bin_pt=0  quantization=Truncate  overflow=Saturate  dbl_ovrd=off  use_behavioral_HDL=off  hw_selection=Fabric  pipelined=off  block_type=addsub
  Convert : xbsIndex_r4/Convert  gui_display_data_type=Boolean  arith_type=Boolean  n_bits=16  bin_pt=14  float_type=Single  exp_bits=8  fraction_bits=24  quantization=Truncate  overflow=Wrap  en=off  latency=0  dbl_ovrd=off  pipeline=off  block_type=convert
  Convert1 : xbsIndex_r4/Convert  gui_display_data_type=Boolean  arith_type=Boolean  n_bits=16  bin_pt=14  float_type=Single  exp_bits=8  fraction_bits=24  quantization=Truncate  overflow=Wrap  en=off  latency=0  dbl_ovrd=off  pipeline=off  block_type=convert
  Dir  Reg : xbsIndex_r4/Register  init=0  rst=off  en=off  dbl_ovrd=off  block_type=register
      settings: xl_area=[10,0,0,0,0,0,0]
  Imp Reg : xbsIndex_r4/Register  init=0  rst=off  en=off  dbl_ovrd=off  block_type=register
      settings: xl_area=[10,0,0,0,0,0,0]
  Inverter : xbsIndex_r4/Inverter  en=off  latency=1  dbl_ovrd=off  block_type=inv
  Kimeneti Reg : xbsIndex_r4/Register  init=0  rst=off  en=on  dbl_ovrd=off  block_type=register
      settings: xl_area=[10,0,0,0,0,0,0]
  Logical : xbsIndex_r4/Logical  logical_function=AND  inputs=2  en=off  latency=0  precision=Full  arith_type=Unsigned  n_bits=16  bin_pt=0  align_bp=on  dbl_ovrd=off  block_type=logical
      settings: xl_use_area=on
  Lépés Neg : xbsIndex_r4/Constant  const=-1  gui_display_data_type=Fixed-point  arith_type=Signed (2's comp)  n_bits=16  bin_pt=0  preci_type=Single  exp_width=8  frac_width=24  explicit_period=off  period=1  equ=P=C  opselect=C  inp2=PCIN>>17  opr=+  inp1=P  carry=CIN  dbl_ovrd=off  block_type=constant
  Lépés Poz : xbsIndex_r4/Constant  const=1  gui_display_data_type=Fixed-point  arith_type=Signed (2's comp)  n_bits=16  bin_pt=0  preci_type=Single  exp_width=8  frac_width=24  explicit_period=off  period=1  equ=P=C  opselect=C  inp2=PCIN>>17  opr=+  inp1=P  carry=CIN  dbl_ovrd=off  block_type=constant
  Mux : xbsIndex_r4/Mux  inputs=2  en=off  latency=0  precision=User Defined  arith_type="Signed  (2's comp)"  n_bits=16  bin_pt=0  quantization=Truncate  overflow=Saturate  dbl_ovrd=off  block_type=mux
  Mux1 : xbsIndex_r4/Mux  inputs=2  en=off  latency=0  precision=User Defined  arith_type=Unsigned  n_bits=1  bin_pt=0  quantization=Truncate  overflow=Saturate  dbl_ovrd=off  block_type=mux
      settings: xl_use_area=on
  Sebesség Reg : xbsIndex_r4/Register  init=0  rst=on  en=on  dbl_ovrd=off  block_type=register
      settings: xl_area=[10,0,0,0,0,0,0]
  Value Counter : Outport
  wires:
  Kimeneti Reg/1 -> Value Counter/1
  Lépés Poz/1 -> Mux/3
  Dir/1 -> Dir  Reg/1
  Inverter/1 -> Logical/2
  Logical/1 -> Convert/1
  Impulse/1 -> Imp Reg/1
  Sebesség Reg/1 -> Kimeneti Reg/1, AddSub/1
  Convert/1 -> Sebesség Reg/3
  SpeedTSimp/1 -> Convert1/1
  Imp Reg/1 -> Logical/1, Inverter/1
  AddSub/1 -> Sebesség Reg/1
  Mux/1 -> AddSub/2
  Lépés Neg/1 -> Mux/2
  Dir  Reg/1 -> " "/1, Mux1/2
  Mux1/1 -> Mux/1
  " "/1 -> Mux1/3
  Convert1/1 -> Kimeneti Reg/2, Sebesség Reg/2
  CserelDir/1 -> Mux1/1

== system IpSDKSebesegEsPozicio/Pozició Szab/SignToUSign ==
  Dir : Inport
  valIn : Inport  Port=2
  Inverter : xbsIndex_r4/Inverter  en=off  latency=0  dbl_ovrd=off  block_type=inv
  Mux : xbsIndex_r4/Mux  inputs=2  en=off  latency=0  precision=Full  arith_type=Unsigned  n_bits=16  bin_pt=0  quantization=Truncate  overflow=Wrap  dbl_ovrd=off  block_type=mux
  val : Outport
  wires:
  Dir/1 -> Mux/1
  valIn/1 -> Inverter/1, Mux/2
  Mux/1 -> val/1
  Inverter/1 -> Mux/3

== system IpSDKSebesegEsPozicio/Sebesség Szab/Mintavételi Jel Generator ==
  STOP : Inport
  Ts : Inport  Port=2
  Convert : xbsIndex_r4/Convert  gui_display_data_type=Boolean  arith_type=Boolean  n_bits=16  bin_pt=14  float_type=Single  exp_bits=8  fraction_bits=24  quantization=Truncate  overflow=Wrap  en=off  latency=0  dbl_ovrd=off  pipeline=off  block_type=convert
  Delay : xbsIndex_r4/Delay  rst=off  infoeditControl=Selection of Reset will increase slice count due to use of real FFs and instead of SRLs  en=off  latency=1  dbl_ovrd=off  reg_retiming=off  block_type=delay
  Inverter : xbsIndex_r4/Inverter  en=off  latency=0  dbl_ovrd=off  block_type=inv
  Kimenet ha STOP=0 : xbsIndex_r4/Logical  logical_function=AND  inputs=2  en=off  latency=0  precision=User Defined  arith_type=Unsigned  n_bits=1  bin_pt=0  align_bp=on  dbl_ovrd=off  block_type=logical
  Periodus vége vagy uj Ts érték : xbsIndex_r4/Logical  logical_function=OR  inputs=2  en=off  latency=0  precision=User Defined  arith_type=Unsigned  n_bits=1  bin_pt=0  align_bp=on  dbl_ovrd=off  block_type=logical
  PeriodusVáge : xbsIndex_r4/Relational  mode=a=b  en=off  latency=0  dbl_ovrd=off  block_type=relational
  Számláló : xbsIndex_r4/Counter  cnt_type=Free Running  cnt_to=Inf  operation=Up  start_count=0  cnt_by_val=1  arith_type=Unsigned  n_bits=32  bin_pt=0  load_pin=off  rst=on  en=off  explicit_period=on  period=1  dbl_ovrd=off  use_behavioral_HDL=off  implementation=Fabric  block_type=counter
  Ts változott : xbsIndex_r4/Relational  mode=a!=b  en=off  latency=0  dbl_ovrd=off  block_type=relational
  Tick : Outport
  wires:
  Számláló/1 -> PeriodusVáge/1
  PeriodusVáge/1 -> Periodus vége vagy uj Ts érték/1, Kimenet ha STOP=0/1
  Kimenet ha STOP=0/1 -> Tick/1
  STOP/1 -> Inverter/1
  Inverter/1 -> Kimenet ha STOP=0/2
  Delay/1 -> Ts változott/2
  Ts/1 -> Ts változott/1, Delay/1, PeriodusVáge/2
  Ts változott/1 -> Periodus vége vagy uj Ts érték/2
  Periodus vége vagy uj Ts érték/1 -> Convert/1
  Convert/1 -> Számláló/1

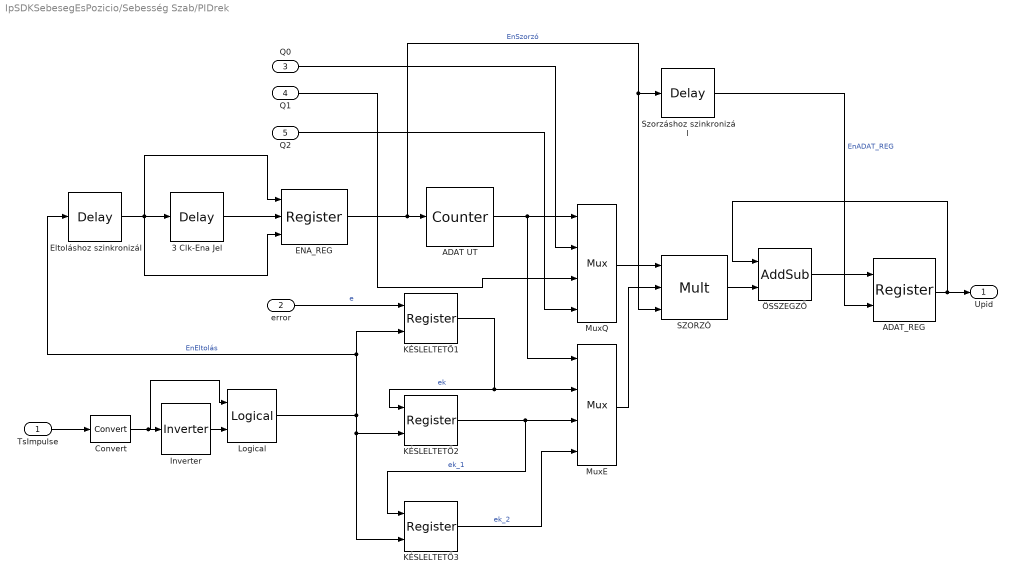
== system IpSDKSebesegEsPozicio/Sebesség Szab/PIDrek ==
  TsImpulse : Inport
  error : Inport  Port=2
  Q0 : Inport  Port=3
  Q1 : Inport  Port=4
  Q2 : Inport  Port=5
  3 Clk-Ena Jel : xbsIndex_r4/Delay  rst=off  infoeditControl=Selection of Reset will increase slice count due to use of real FFs and instead of SRLs  en=off  latency=3  dbl_ovrd=off  reg_retiming=off  block_type=delay
  ADAT UT : xbsIndex_r4/Counter  cnt_type=Count Limited  cnt_to=2  operation=Up  start_count=0  cnt_by_val=1  arith_type=Unsigned  n_bits=2  bin_pt=0  load_pin=off  rst=off  en=on  explicit_period=on  period=1  dbl_ovrd=off  use_behavioral_HDL=off  implementation=Fabric  block_type=counter
      settings: xl_area=[100,0,0,0,0,0,0]
  ADAT_REG : xbsIndex_r4/Register  init=0  rst=off  en=on  dbl_ovrd=off  block_type=register
      settings: xl_area=[100,0,0,0,0,0,0]
  Convert : xbsIndex_r4/Convert  gui_display_data_type=Boolean  arith_type=Boolean  n_bits=16  bin_pt=14  float_type=Single  exp_bits=8  fraction_bits=24  quantization=Truncate  overflow=Wrap  en=off  latency=0  dbl_ovrd=off  pipeline=off  block_type=convert
  ENA_REG : xbsIndex_r4/Register  init=0  rst=on  en=on  dbl_ovrd=off  block_type=register
  Eltoláshoz szinkronizál : xbsIndex_r4/Delay  rst=off  infoeditControl=Selection of Reset will increase slice count due to use of real FFs and instead of SRLs  en=off  latency=1  dbl_ovrd=off  reg_retiming=off  block_type=delay
  Inverter : xbsIndex_r4/Inverter  en=off  latency=1  dbl_ovrd=off  block_type=inv
  KÉSLELTETŐ1 : xbsIndex_r4/Register  init=0  rst=off  en=on  dbl_ovrd=off  block_type=register
      settings: xl_area=[100,0,0,0,0,0,0]
  KÉSLELTETŐ2 : xbsIndex_r4/Register  init=0  rst=off  en=on  dbl_ovrd=off  block_type=register
      settings: xl_area=[100,0,0,0,0,0,0]
  KÉSLELTETŐ3 : xbsIndex_r4/Register  init=0  rst=off  en=on  dbl_ovrd=off  block_type=register
  Logical : xbsIndex_r4/Logical  logical_function=AND  inputs=2  en=off  latency=0  precision=Full  arith_type=Unsigned  n_bits=16  bin_pt=0  align_bp=on  dbl_ovrd=off  block_type=logical
  MuxE : xbsIndex_r4/Mux  inputs=3  en=off  latency=0  precision=User Defined  arith_type="Signed  (2's comp)"  n_bits=16  bin_pt=0  quantization=Truncate  overflow=Saturate  dbl_ovrd=off  block_type=mux
      settings: xl_use_area=on  xl_area=[1,0,0,0,0,0,0]
  MuxQ : xbsIndex_r4/Mux  inputs=3  en=off  latency=0  precision=User Defined  arith_type="Signed  (2's comp)"  n_bits=16  bin_pt=0  quantization=Truncate  overflow=Saturate  dbl_ovrd=off  block_type=mux
      settings: xl_area=[1,0,0,0,0,0,0]
  SZORZÓ : xbsIndex_r4/Mult  precision=User Defined  arith_type="Signed  (2's comp)"  n_bits=17  bin_pt=0  quantization=Truncate  overflow=Saturate  en=on  latency=1  dbl_ovrd=off  use_behavioral_HDL=off  opt=Area  use_embedded=on  optimum_pipeline=off  pipeline=on  use_rpm=on  placement_style=Triangular  block_type=mult
  Szorzáshoz szinkronizál : xbsIndex_r4/Delay  rst=off  infoeditControl=Selection of Reset will increase slice count due to use of real FFs and instead of SRLs  en=off  latency=1  dbl_ovrd=off  reg_retiming=off  block_type=delay
  ÖSSZEGZŐ : xbsIndex_r4/AddSub  mode=Addition  use_carryin=off  use_carryout=off  en=off  latency=0  precision=User Defined  arith_type="Signed  (2's comp)"  n_bits=17  bin_pt=0  quantization=Truncate  overflow=Saturate  dbl_ovrd=off  use_behavioral_HDL=off  hw_selection=Fabric  pipelined=off  block_type=addsub
      settings: xl_area=[100,0,0,0,0,0,0]
  Upid : Outport
  wires:
  MuxQ/1 -> SZORZÓ/1
  MuxE/1 -> SZORZÓ/2
  KÉSLELTETŐ2/1 -> KÉSLELTETŐ3/1, MuxE/3  "ek_1"
  ÖSSZEGZŐ/1 -> ADAT_REG/1
  3 Clk-Ena Jel/1 -> ENA_REG/2
  SZORZÓ/1 -> ÖSSZEGZŐ/2
  Szorzáshoz szinkronizál/1 -> ADAT_REG/2  "EnADAT_REG"
  ADAT_REG/1 -> Upid/1, ÖSSZEGZŐ/1
  ADAT UT/1 -> MuxE/1, MuxQ/1
  ENA_REG/1 -> Szorzáshoz szinkronizál/1, SZORZÓ/3, ADAT UT/1  "EnSzorzó"
  Q2/1 -> MuxQ/4
  KÉSLELTETŐ3/1 -> MuxE/4  "ek_2"
  Eltoláshoz szinkronizál/1 -> 3 Clk-Ena Jel/1, ENA_REG/3, ENA_REG/1
  KÉSLELTETŐ1/1 -> MuxE/2, KÉSLELTETŐ2/1  "ek"
  Q0/1 -> MuxQ/2
  Q1/1 -> MuxQ/3
  Inverter/1 -> Logical/2
  TsImpulse/1 -> Convert/1
  Logical/1 -> KÉSLELTETŐ3/2, KÉSLELTETŐ2/2, Eltoláshoz szinkronizál/1, KÉSLELTETŐ1/2  "EnEltolás"
  error/1 -> KÉSLELTETŐ1/1  "e"
  Convert/1 -> Inverter/1, Logical/1

== system IpSDKSebesegEsPozicio/Sebesség Szab/PWM ==
  Duty : Inport
  en : Inport  Port=2
  96%MaxKitöltés : xbsIndex_r4/Constant  const=15563  gui_display_data_type=Fixed-point  arith_type=Unsigned  n_bits=16  bin_pt=0  preci_type=Single  exp_width=8  frac_width=24  explicit_period=off  period=1  equ=P=C  opselect=C  inp2=PCIN>>17  opr=+  inp1=P  carry=CIN  dbl_ovrd=off  block_type=constant
  Counter : xbsIndex_r4/Counter  cnt_type=Free Running  cnt_to=Inf  operation=Up  start_count=0  cnt_by_val=1  arith_type=Unsigned  n_bits=16  bin_pt=0  load_pin=off  rst=on  en=on  explicit_period=off  period=2*10^-2  dbl_ovrd=off  use_behavioral_HDL=off  implementation=Fabric  block_type=counter
  Kitöltés vége : xbsIndex_r4/Relational  mode=a>b  en=off  latency=0  dbl_ovrd=off  block_type=relational
  Kitöltés korlátozása : xbsIndex_r4/Relational  mode=a>b  en=off  latency=0  dbl_ovrd=off  block_type=relational
  Logical : xbsIndex_r4/Logical  logical_function=AND  inputs=2  en=off  latency=0  precision=User Defined  arith_type=Unsigned  n_bits=1  bin_pt=0  align_bp=on  dbl_ovrd=off  block_type=logical
  Mux : xbsIndex_r4/Mux  inputs=2  en=off  latency=0  precision=User Defined  arith_type=Unsigned  n_bits=16  bin_pt=0  quantization=Truncate  overflow=Wrap  dbl_ovrd=off  block_type=mux
  Periodus vége : xbsIndex_r4/Relational  mode=a=b  en=off  latency=0  dbl_ovrd=off  block_type=relational
  Periodus Reg : xbsIndex_r4/Constant  const=16383  gui_display_data_type=Fixed-point  arith_type=Unsigned  n_bits=17  bin_pt=0  preci_type=Single  exp_width=8  frac_width=24  explicit_period=off  period=1  equ=P=C  opselect=C  inp2=PCIN>>17  opr=+  inp1=P  carry=CIN  dbl_ovrd=off  block_type=constant
  Shift : xbsIndex_r4/Shift  shift_dir=Right  shift_bits=2  en=off  latency=0  precision=User Defined  arith_type="Signed  (2's comp)"  n_bits=16  bin_pt=0  quantization=Truncate  overflow=Saturate  dbl_ovrd=off  block_type=shift
  PWM : Outport
  wires:
  Counter/1 -> Periodus vége/1, Kitöltés vége/2
  Periodus vége/1 -> Counter/1
  en/1 -> Logical/2, Counter/2
  Kitöltés vége/1 -> Logical/1
  Logical/1 -> PWM/1
  Duty/1 -> Shift/1
  Periodus Reg/1 -> Periodus vége/2
  96%MaxKitöltés/1 -> Mux/2, Kitöltés korlátozása/1
  Mux/1 -> Kitöltés vége/1
  Kitöltés korlátozása/1 -> Mux/1
  Shift/1 -> Mux/3, Kitöltés korlátozása/2

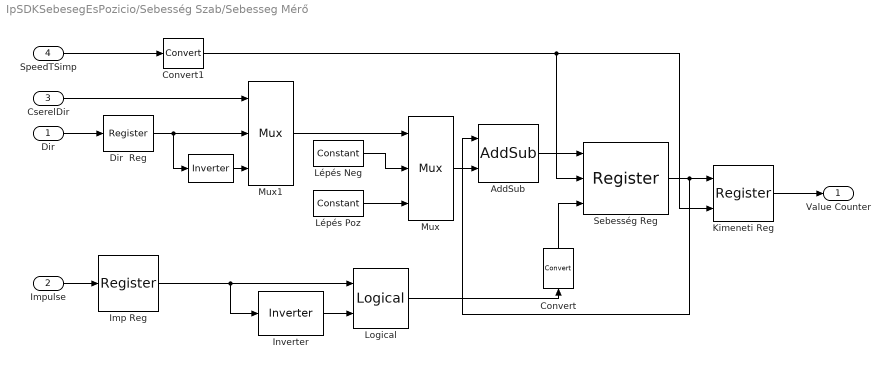
== system IpSDKSebesegEsPozicio/Sebesség Szab/Sebesseg Mérő ==
  Dir : Inport
  Impulse : Inport  Port=2
  CserelDir : Inport  Port=3
  SpeedTSimp : Inport  Port=4
  " " : xbsIndex_r4/Inverter  en=off  latency=0  dbl_ovrd=off  block_type=inv
      settings: xl_area=[10,0,0,0,0,0,0]
  AddSub : xbsIndex_r4/AddSub  mode=Addition  use_carryin=off  use_carryout=off  en=off  latency=0  precision=User Defined  arith_type="Signed  (2's comp)"  n_bits=16  bin_pt=0  quantization=Truncate  overflow=Saturate  dbl_ovrd=off  use_behavioral_HDL=off  hw_selection=Fabric  pipelined=off  block_type=addsub
  Convert : xbsIndex_r4/Convert  gui_display_data_type=Boolean  arith_type=Boolean  n_bits=16  bin_pt=14  float_type=Single  exp_bits=8  fraction_bits=24  quantization=Truncate  overflow=Wrap  en=off  latency=0  dbl_ovrd=off  pipeline=off  block_type=convert
  Convert1 : xbsIndex_r4/Convert  gui_display_data_type=Boolean  arith_type=Boolean  n_bits=16  bin_pt=14  float_type=Single  exp_bits=8  fraction_bits=24  quantization=Truncate  overflow=Wrap  en=off  latency=0  dbl_ovrd=off  pipeline=off  block_type=convert
  Dir  Reg : xbsIndex_r4/Register  init=0  rst=off  en=off  dbl_ovrd=off  block_type=register
      settings: xl_area=[10,0,0,0,0,0,0]
  Imp Reg : xbsIndex_r4/Register  init=0  rst=off  en=off  dbl_ovrd=off  block_type=register
      settings: xl_area=[10,0,0,0,0,0,0]
  Inverter : xbsIndex_r4/Inverter  en=off  latency=1  dbl_ovrd=off  block_type=inv
  Kimeneti Reg : xbsIndex_r4/Register  init=0  rst=off  en=on  dbl_ovrd=off  block_type=register
      settings: xl_area=[10,0,0,0,0,0,0]
  Logical : xbsIndex_r4/Logical  logical_function=AND  inputs=2  en=off  latency=0  precision=Full  arith_type=Unsigned  n_bits=16  bin_pt=0  align_bp=on  dbl_ovrd=off  block_type=logical
      settings: xl_use_area=on
  Lépés Neg : xbsIndex_r4/Constant  const=-1  gui_display_data_type=Fixed-point  arith_type=Signed (2's comp)  n_bits=16  bin_pt=0  preci_type=Single  exp_width=8  frac_width=24  explicit_period=off  period=1  equ=P=C  opselect=C  inp2=PCIN>>17  opr=+  inp1=P  carry=CIN  dbl_ovrd=off  block_type=constant
  Lépés Poz : xbsIndex_r4/Constant  const=1  gui_display_data_type=Fixed-point  arith_type=Signed (2's comp)  n_bits=16  bin_pt=0  preci_type=Single  exp_width=8  frac_width=24  explicit_period=off  period=1  equ=P=C  opselect=C  inp2=PCIN>>17  opr=+  inp1=P  carry=CIN  dbl_ovrd=off  block_type=constant
  Mux : xbsIndex_r4/Mux  inputs=2  en=off  latency=0  precision=User Defined  arith_type="Signed  (2's comp)"  n_bits=16  bin_pt=0  quantization=Truncate  overflow=Saturate  dbl_ovrd=off  block_type=mux
  Mux1 : xbsIndex_r4/Mux  inputs=2  en=off  latency=0  precision=User Defined  arith_type=Unsigned  n_bits=1  bin_pt=0  quantization=Truncate  overflow=Saturate  dbl_ovrd=off  block_type=mux
      settings: xl_use_area=on
  Sebesség Reg : xbsIndex_r4/Register  init=0  rst=on  en=on  dbl_ovrd=off  block_type=register
      settings: xl_area=[10,0,0,0,0,0,0]
  Value Counter : Outport
  wires:
  Kimeneti Reg/1 -> Value Counter/1
  Lépés Poz/1 -> Mux/3
  Dir/1 -> Dir  Reg/1
  Inverter/1 -> Logical/2
  Logical/1 -> Convert/1
  Impulse/1 -> Imp Reg/1
  Sebesség Reg/1 -> Kimeneti Reg/1, AddSub/1
  Convert/1 -> Sebesség Reg/3
  SpeedTSimp/1 -> Convert1/1
  Imp Reg/1 -> Logical/1, Inverter/1
  AddSub/1 -> Sebesség Reg/1
  Mux/1 -> AddSub/2
  Lépés Neg/1 -> Mux/2
  Dir  Reg/1 -> " "/1, Mux1/2
  Mux1/1 -> Mux/1
  " "/1 -> Mux1/3
  Convert1/1 -> Kimeneti Reg/2, Sebesség Reg/2
  CserelDir/1 -> Mux1/1

== system IpSDKSebesegEsPozicio/Sebesség Szab/SignToUSign ==
  Dir : Inport
  valIn : Inport  Port=2
  Inverter : xbsIndex_r4/Inverter  en=off  latency=0  dbl_ovrd=off  block_type=inv
  Mux : xbsIndex_r4/Mux  inputs=2  en=off  latency=0  precision=Full  arith_type=Unsigned  n_bits=16  bin_pt=0  quantization=Truncate  overflow=Wrap  dbl_ovrd=off  block_type=mux
  val : Outport
  wires:
  Dir/1 -> Mux/1
  valIn/1 -> Inverter/1, Mux/2
  Mux/1 -> val/1
  Inverter/1 -> Mux/3
